simulink model "order_reduction_model"  (R2021a)
settings: Solver=FixedStepAuto  StartTime=0.0  StopTime=conf.cycle.stop  FixedStep=conf.time.step  RelTol=1e-3
InitFcn:
  | full_model_init;
  | load([pwd '\Data\pca_results.mat']);
values from neighbouring files (symbols this model uses):
  A = AB(1:10,:)    [order_reduction_script.m]
  B = AB(11:12,:)    [order_reduction_script.m]
  cellsP = conf.cells.p    [full_model_init.m]
  cellsS = conf.modules.x*conf.modules.y*conf.cells.s    [full_model_init.m]
  cellsTot = cellsS*cellsP    [full_model_init.m]
  elecC1 = C1_matrix*elecCellCap/cellCapGiant    [full_model_init.m]
  elecCellCap = 60    [full_model_init.m]
  elecInitSOC = (1 - variation)*socAve + 2*variation*socAve*rand(cellsS,cellsP)    [full_model_init.m]
  elecLoadDenomInds = 0    [full_model_init.m]
  elecLoadTerm12Inds = 0    [full_model_init.m]
  elecLoadTerm1Inds = 0    [full_model_init.m]
  elecLoadTerm2Inds = 0    [full_model_init.m]
  elecLoadTerm3Inds = 0    [full_model_init.m]
  elecOCV = Em_matrix    [full_model_init.m]
  elecR0 = R1_matrix*cellCapGiant/elecCellCap    [full_model_init.m]
  elecR1 = R2_matrix*cellCapGiant/elecCellCap    [full_model_init.m]
  elecSOCBreak = SOC_breakpoints    [full_model_init.m]
  elecTempBreak = Temp_breakpoints    [full_model_init.m]
  maxFlow = min([maxFlowX maxFlowY])    [full_model_init.m]
  mdotDistX = mdotDistX*flowMult    [full_model_init.m]
  mdotDistY = mdotDistY*flowMult    [full_model_init.m]
  tempAmb = conf.bound.amb    [full_model_init.m]    (also in order_reduction_script.m = data.tempAmb)
  tempTarget = 25    [full_model_init.m]
  thermCellVols = (thermHeatInds ~= 0)    [full_model_init.m]
  thermHeatCellToVol = 1/(conf.regions.l*conf.regions.w*conf.regions.t)    [full_model_init.m]
  thermTempInds = zeros(conf.regions.l*conf.regions.w*conf.regions.t,1,cellsS*cellsP)    [full_model_init.m]
  vehAf = 3.15    [full_model_init.m]
  vehCd = 0.28    [full_model_init.m]
  vehM = 2565    [full_model_init.m]
  vehPowerMult = modelEnergy/packEnergy    [full_model_init.m]
undefined symbols (not defined in the file or in its folder): conf, loadDenomInds, loadTerm12Inds, loadTerm1Inds, loadTerm2Inds, loadTerm3Inds, parallelCells, radAirVelBreakPoints, radCoolFlowBreakPoints, radNomFlowMatrix, refAirVelBreakPoints, refCoolFlowBreakPoints, refCoolInTempBreakPoints, refTempOutMatrix, seriesCells, thermDims
libraries: visionstatistics x1
settings Model: NumberOfSteps=100  Creator=sjtho  LastModifiedBy=sjtho
settings OptimizationCC: OptimizeBlockIOStorage=off  OptimizeDataStoreBuffers=off  BusAssignmentInplaceUpdate=off
settings DebuggingCC: UniqueDataStoreMsg=error  SFUnexpectedBacktrackingDiag=warning  SFNoUnconditionalDefaultTransitionDiag=warning
settings RTWCC: GenerateReport=on  BuildConfiguration=Debug  LaunchReport=on
settings CodeAppCC: ForceParamTrailComments=on  MATLABSourceComments=on  EnableCustomComments=on
settings GRTTargetCC: CombineSignalStateStructs=on  SupportVariableSizeSignals=on  MultiInstanceErrorCode=Warning

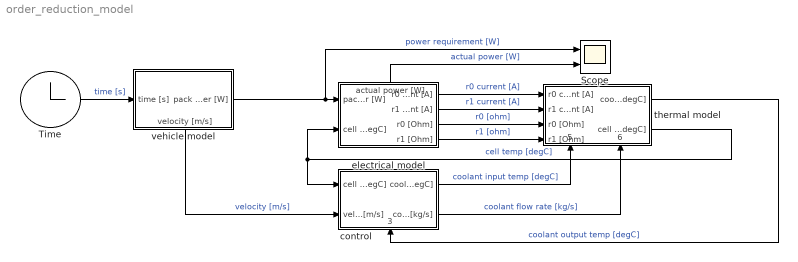
== system order_reduction_model ==
  Scope : Scope  NumInputPorts=2
  Time : Clock
  control : Subsystem
      settings: PortSchema="{\"entries\":[{\"content\":{\"sides\":[{\"content\":{\"connectorIds\":[\"In1\",\"In2\"]},\"type\":\"ConnectorPlacement.EquallySpacedRectSide\",\"uuid\":\"22f80eaa-bb46-4281-9ec1-3970c1bac2a3\"},{\"content\":{\"connectorIds\":[\"Out1\",\"Out2\"],\"side\":\"RIGHT\"},\"type\":\"ConnectorPlacement.EquallySpacedRectSide\",\"uuid\":\"e76f71c5-d41f-442d-b655-b3bc32395443\"},{\"content\":{\"connectorIds\":[],\"side\":\"TOP\"},\"type\":\"ConnectorPlacement.EquallySpacedRectSide\",\"uuid\":\"e3a9d903-5780-49ee-b4b3-f001d4a3722b\"},{\"content\":{\"connectorIds\":[\"In3\"],\"side\":\"BOTTOM\"},\"type\":\"ConnectorPlacement.EquallySpacedRectSide\",\"uuid\":\"8a36595f-00ae-4362-a59c-271e32328d9e\"}]},\"type\":\"ConnectorPlacement.EquallySpacedConnector\",\"uuid\":\"d37af0d9-ec54-4f0d-b375-47d72f1b804c\"}],\"packageUris\":[\"http://schema.mathworks.com/mf0/Connector/R2020b\"],\"version\":\"1.0\"}"
      mask Display: disp(['Control and ' newline 'Cooling'])
  electrical model : Subsystem
      settings: PortSchema="{\"entries\":[{\"content\":{\"sides\":[{\"content\":{\"connectorIds\":[\"In1\",\"In2\"]},\"type\":\"ConnectorPlacement.EquallySpacedRectSide\",\"uuid\":\"4f52e6ae-bc3b-4951-b08d-fa2762ef8feb\"},{\"content\":{\"connectorIds\":[\"Out1\",\"Out2\",\"Out3\",\"Out4\"],\"side\":\"RIGHT\"},\"type\":\"ConnectorPlacement.EquallySpacedRectSide\",\"uuid\":\"4046dfc3-1b24-4486-8fe3-cced4e699fd9\"},{\"content\":{\"connectorIds\":[\"Out5\"],\"side\":\"TOP\"},\"type\":\"ConnectorPlacement.EquallySpacedRectSide\",\"uuid\":\"da108a30-fb00-422c-8122-750755c2660a\"}]},\"type\":\"ConnectorPlacement.EquallySpacedConnector\",\"uuid\":\"4753e952-e769-49fa-907f-6d09e5e535ba\"}],\"packageUris\":[\"http://schema.mathworks.com/mf0/Connector/R2020b\"],\"version\":\"1.0\"}"
      mask Display: disp('Electrical Model')
  thermal model : Subsystem
      settings: PortSchema="{\"entries\":[{\"content\":{\"sides\":[{\"content\":{\"connectorIds\":[\"In1\",\"In2\",\"In3\",\"In4\"]},\"type\":\"ConnectorPlacement.EquallySpacedRectSide\",\"uuid\":\"85abd361-fdf9-4e50-9692-c6cfc682c3ac\"},{\"content\":{\"connectorIds\":[\"Out1\",\"Out2\"],\"side\":\"RIGHT\"},\"type\":\"ConnectorPlacement.EquallySpacedRectSide\",\"uuid\":\"50be5dc9-6285-4d3d-a0f1-610cf70c20d6\"},{\"content\":{\"connectorIds\":[],\"side\":\"TOP\"},\"type\":\"ConnectorPlacement.EquallySpacedRectSide\",\"uuid\":\"1bb98c42-8893-43bf-953b-d262aeaa61fe\"},{\"content\":{\"connectorIds\":[\"In5\",\"In6\"],\"side\":\"BOTTOM\"},\"type\":\"ConnectorPlacement.EquallySpacedRectSide\",\"uuid\":\"83d18484-4c30-41fd-9096-006931d5d21f\"}]},\"type\":\"ConnectorPlacement.EquallySpacedConnector\",\"uuid\":\"8afb65a4-2410-4c66-9cd3-3c36ab441c83\"}],\"packageUris\":[\"http://schema.mathworks.com/mf0/Connector/R2020b\"],\"version\":\"1.0\"}"
      mask Display: disp('Thermal Model')
  vehicle model : Subsystem
      settings: PortSchema="{\"entries\":[{\"content\":{\"sides\":[{\"content\":{\"connectorIds\":[\"In1\"]},\"type\":\"ConnectorPlacement.EquallySpacedRectSide\",\"uuid\":\"cf313784-55fc-4068-b83a-27fead484f77\"},{\"content\":{\"connectorIds\":[\"Out1\"],\"side\":\"RIGHT\"},\"type\":\"ConnectorPlacement.EquallySpacedRectSide\",\"uuid\":\"2b8b7e96-e7dc-4089-926d-80148fade29f\"},{\"content\":{\"connectorIds\":[],\"side\":\"TOP\"},\"type\":\"ConnectorPlacement.EquallySpacedRectSide\",\"uuid\":\"332287a3-327f-4bf8-9290-89809e483fea\"},{\"content\":{\"connectorIds\":[\"Out2\"],\"side\":\"BOTTOM\"},\"type\":\"ConnectorPlacement.EquallySpacedRectSide\",\"uuid\":\"f07f6670-fe7e-40c0-9cd8-41a00d5f5993\"}]},\"type\":\"ConnectorPlacement.EquallySpacedConnector\",\"uuid\":\"6bd39f86-8f76-4883-86c4-8a861857bd9f\"}],\"packageUris\":[\"http://schema.mathworks.com/mf0/Connector/R2020b\"],\"version\":\"1.0\"}"
      mask Display: disp('Vehicle Model')
  wires:
  Time/1 -> vehicle model/1(time [s])  "time [s]"
  vehicle model/1(pack power [W]) -> Scope/1, electrical model/1(pack power [W])  "power requirement [W]"
  control/1(coolant input temp [degC]) -> thermal model/5(coolant input temp [degC])  "coolant input temp [degC]"
  thermal model/1(coolant output temp [degC]) -> control/3(coolant output temp [degC])  "coolant output temp [degC]"
  electrical model/1(r0 current [A]) -> thermal model/1(r0 current [A])  "r0 current [A]"
  electrical model/2(r1 current [A]) -> thermal model/2(r1 current [A])  "r1 current [A]"
  electrical model/3(r0 [Ohm]) -> thermal model/3(r0 [Ohm])  "r0 [ohm]"
  electrical model/4(r1 [Ohm]) -> thermal model/4(r1 [Ohm])  "r1 [ohm]"
  thermal model/2(cell temp [degC]) -> electrical model/2(cell temp [degC]), control/1(cell temp [degC])  "cell temp [degC]"
  electrical model/5(actual power [W]) -> Scope/2  "actual power [W]"
  vehicle model/2(velocity [m/s]) -> control/2(velocity [m/s])  "velocity [m/s]"
  control/2(coolant flow rate [kg/s]) -> thermal model/6(coolant flow rate [kg/s])  "coolant flow rate [kg/s]"

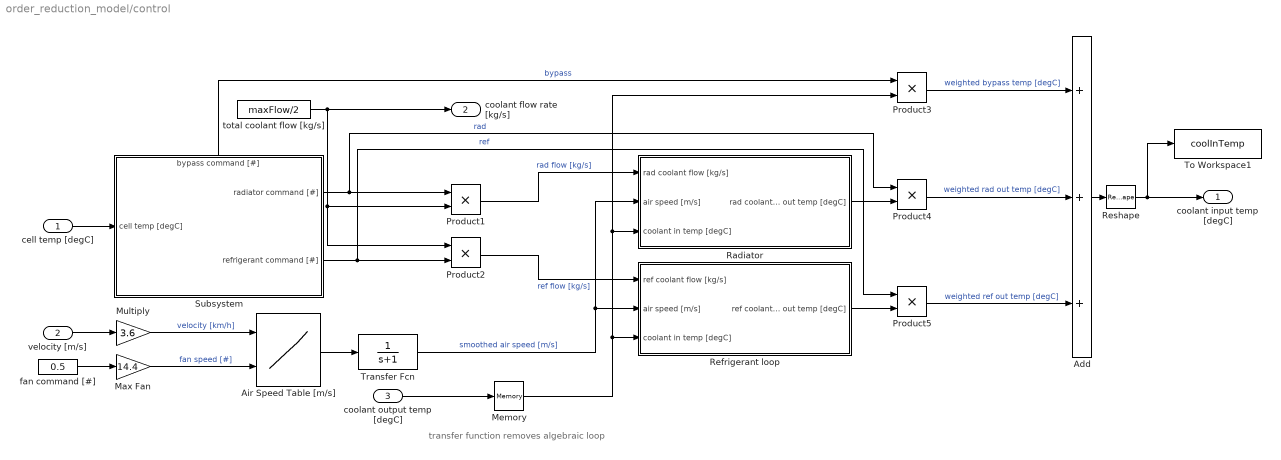
== system order_reduction_model/control ==
  note: transfer function removes algebraic loop
  cell temp [degC] : Inport
  velocity [m/s] : Inport  Port=2
  coolant output temp [degC] : Inport  Port=3
  Add : Sum  Inputs=+++
  Air Speed Table [m/s] : Lookup_n-D  BreakpointsForDimension1=[0 40 90 110 150 180 198]  BreakpointsForDimension2=[0 14.4]  IndexSearchMethod=Linear search  BeginIndexSearchUsingPreviousIndexResult=on  Table=[0 0.8 2.2 2.7 3.6 4.1 4.6; 1.5 2.3 3.2 3.5 4.3 4.8 5.1]'  InternalRulePriority=Speed  RndMeth=Simplest  InputSameDT=on
      settings: InputPortMap=u0,u1
  Max Fan : Gain  Gain=14.4
  Memory : Memory  InitialCondition=tempAmb + conf.bound.initBias
  Multiply : Gain  Gain=3.6
  Product{1..5} (5 alike) : Product
  Radiator : Subsystem
  Refrigerant loop : Subsystem
  Reshape : Reshape  OutputDimensionality=Customize  OutputDimensions=1
  Subsystem : Subsystem
      settings: PortSchema="{\"entries\":[{\"content\":{\"sides\":[{\"content\":{\"connectorIds\":[\"In1\"]},\"type\":\"ConnectorPlacement.EquallySpacedRectSide\",\"uuid\":\"39caf9d2-37e9-4ddb-8f89-28cdec2ac0f1\"},{\"content\":{\"connectorIds\":[\"Out1\",\"Out2\"],\"side\":\"RIGHT\"},\"type\":\"ConnectorPlacement.EquallySpacedRectSide\",\"uuid\":\"3cbc02da-b039-4e1d-b42e-efc08ec78021\"},{\"content\":{\"connectorIds\":[\"Out3\"],\"side\":\"TOP\"},\"type\":\"ConnectorPlacement.EquallySpacedRectSide\",\"uuid\":\"b4b3f97e-dd64-49e3-8c52-9947fb1a0732\"}]},\"type\":\"ConnectorPlacement.EquallySpacedConnector\",\"uuid\":\"4860c07b-2c7d-4cd4-976e-5c2ba4e5db64\"}],\"packageUris\":[\"http://schema.mathworks.com/mf0/Connector/R2020b\"],\"version\":\"1.0\"}"
  To Workspace1 : ToWorkspace  VariableName=coolInTemp  SaveFormat=Timeseries  SampleTime=conf.time.sample
  Transfer Fcn : TransferFcn  Denominator=[1 1]
  fan command [#] : Constant  Value=0.5
  total coolant flow [kg/s] : Constant  Value=maxFlow/2
  coolant input temp [degC] : Outport
  coolant flow rate [kg/s] : Outport  Port=2
  wires:
  Max Fan/1 -> Air Speed Table [m/s]/2  "fan speed [#]"
  velocity [m/s]/1 -> Multiply/1
  fan command [#]/1 -> Max Fan/1
  Multiply/1 -> Air Speed Table [m/s]/1  "velocity [km/h]"
  Air Speed Table [m/s]/1 -> Transfer Fcn/1
  cell temp [degC]/1 -> Subsystem/1(cell temp [degC])
  Subsystem/1(radiator command [#]) -> Product1/1, Product4/1  "rad"
  Subsystem/2(refrigerant command [#]) -> Product5/1, Product2/2  "ref"
  Product1/1 -> Radiator/1(rad coolant flow [kg/s])  "rad flow [kg/s]"
  Product2/1 -> Refrigerant loop/1(ref coolant flow [kg/s])  "ref flow [kg/s]"
  Transfer Fcn/1 -> Radiator/2(air speed [m/s]), Refrigerant loop/2(air speed [m/s])  "smoothed air speed [m/s]"
  coolant output temp [degC]/1 -> Memory/1
  Refrigerant loop/1(ref coolant out temp [degC]) -> Product5/2
  Radiator/1(rad coolant out temp [degC]) -> Product4/2
  Product4/1 -> Add/2  "weighted rad out temp [degC]"
  Product5/1 -> Add/3  "weighted ref out temp [degC]"
  Product3/1 -> Add/1  "weighted bypass temp [degC]"
  Subsystem/3(bypass command [#]) -> Product3/1  "bypass"
  total coolant flow [kg/s]/1 -> Product2/1, Product1/2, coolant flow rate [kg/s]/1
  Memory/1 -> Product3/2, Radiator/3(coolant in temp [degC]), Refrigerant loop/3(coolant in temp [degC])
  Add/1 -> Reshape/1
  Reshape/1 -> To Workspace1/1, coolant input temp [degC]/1

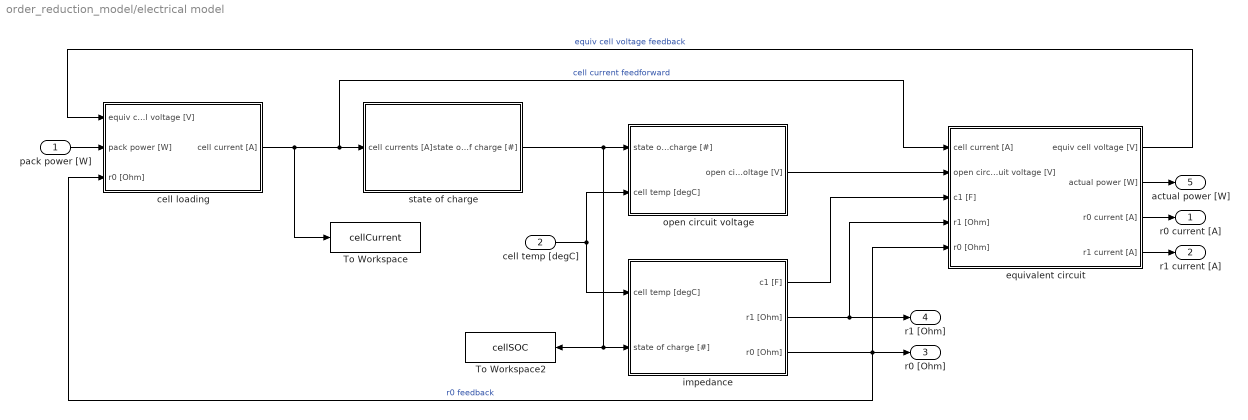
== system order_reduction_model/electrical model ==
  pack power [W] : Inport
  cell temp [degC] : Inport  Port=2
  To Workspace : ToWorkspace  VariableName=cellCurrent  SaveFormat=Timeseries  SampleTime=conf.time.sample
  To Workspace2 : ToWorkspace  VariableName=cellSOC  SaveFormat=Timeseries  SampleTime=conf.time.sample
  cell loading : Subsystem
  equivalent circuit : Subsystem
  impedance : Subsystem
  open circuit voltage : Subsystem
  state of charge : Subsystem
  r0 current [A] : Outport
  r1 current [A] : Outport  Port=2
  r0 [Ohm] : Outport  Port=3
  r1 [Ohm] : Outport  Port=4
  actual power [W] : Outport  Port=5
  wires:
  cell loading/1(cell current [A]) -> To Workspace/1, state of charge/1(cell currents [A]), equivalent circuit/1(cell current [A])  "cell current feedforward"
  cell temp [degC]/1 -> open circuit voltage/2(cell temp [degC]), impedance/1(cell temp [degC])
  state of charge/1(state of charge [#]) -> open circuit voltage/1(state of charge [#]), To Workspace2/1, impedance/2(state of charge [#])
  open circuit voltage/1(open circuit voltage [V]) -> equivalent circuit/2(open circuit voltage [V])
  equivalent circuit/2(actual power [W]) -> actual power [W]/1
  equivalent circuit/3(r0 current [A]) -> r0 current [A]/1
  equivalent circuit/4(r1 current [A]) -> r1 current [A]/1
  equivalent circuit/1(equiv cell voltage [V]) -> cell loading/1(equiv cell voltage [V])  "equiv cell voltage feedback"
  pack power [W]/1 -> cell loading/2(pack power [W])
  impedance/1(c1 [F]) -> equivalent circuit/3(c1 [F])
  impedance/2(r1 [Ohm]) -> r1 [Ohm]/1, equivalent circuit/4(r1 [Ohm])
  impedance/3(r0 [Ohm]) -> r0 [Ohm]/1, cell loading/3(r0 [Ohm]), equivalent circuit/5(r0 [Ohm])  "r0 feedback"

== system order_reduction_model/thermal model ==
  r0 current [A] : Inport
  r1 current [A] : Inport  Port=2
  r0 [Ohm] : Inport  Port=3
  r1 [Ohm] : Inport  Port=4
  coolant input temp [degC] : Inport  Port=5
  coolant flow rate [kg/s] : Inport  Port=6
  Subsystem : Subsystem
      mask Display: disp('Coolant Output Temp');
  cell temp : Subsystem
      mask Display: disp('Cell Temp')
  heat generation : Subsystem
      mask Display: disp('Heat Generation')
  coolant output temp [degC] : Outport
  cell temp [degC] : Outport  Port=2
  wires:
  coolant input temp [degC]/1 -> cell temp/2(coolant input temp [degC])
  r0 current [A]/1 -> heat generation/1(r0 current [A])
  r1 current [A]/1 -> heat generation/2(r1 current [A])
  r0 [Ohm]/1 -> heat generation/3(r0 [Ohm])
  r1 [Ohm]/1 -> heat generation/4(r1 [Ohm])
  heat generation/1(total heat generation [W]) -> cell temp/1(net heat gain [W])  "total heat generation [W]"
  cell temp/1(cell temp [degC]) -> cell temp [degC]/1
  Subsystem/1(coolant output temp [degC]) -> coolant output temp [degC]/1
  cell temp/2(vol temp [degC]) -> Subsystem/2(volume temp [degC])  "volume temp [degC]"
  coolant flow rate [kg/s]/1 -> Subsystem/1(coolant flow rate [kg/s])

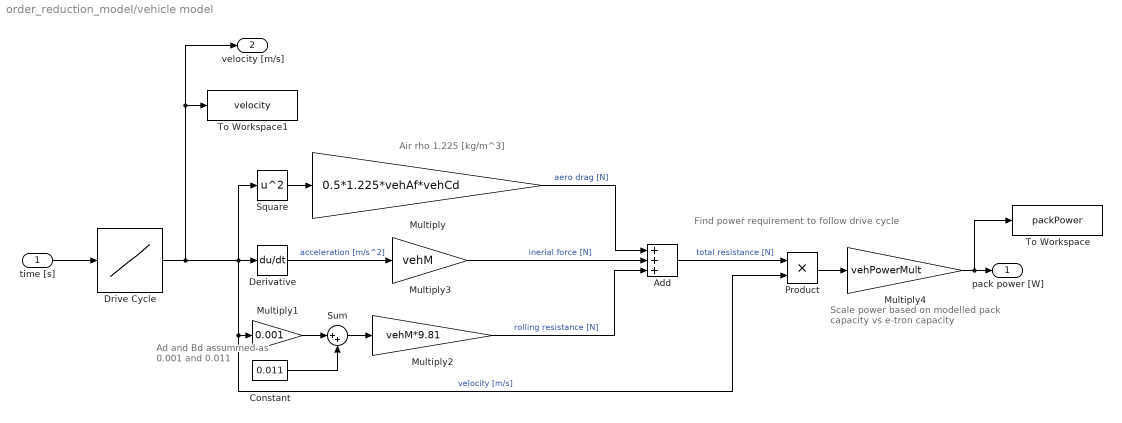
== system order_reduction_model/vehicle model ==
  note: Scale power based on modelled pack capacity vs e-tron capacity
  note: Ad and Bd assummed as 0.001 and 0.011
  note: Air rho 1.225 [kg/m^3]
  note: Find power requirement to follow drive cycle
  time [s] : Inport
  Add : Sum  Inputs=+++
  Constant : Constant  Value=0.011
  Derivative : Derivative
  Drive Cycle : Lookup_n-D  NumberOfTableDimensions=1  BreakpointsForDimension1=conf.cycle.time  Table=conf.cycle.vel  InterpMethod=Cubic spline  InternalRulePriority=Speed  RndMeth=Simplest  InputSameDT=on
  Multiply : Gain  Gain=0.5*1.225*vehAf*vehCd
  Multiply1 : Gain  Gain=0.001
  Multiply2 : Gain  Gain=vehM*9.81
  Multiply3 : Gain  Gain=vehM
  Multiply4 : Gain  Gain=vehPowerMult
  Product : Product
  Square : Math  Operator=square  SaturateOnIntegerOverflow=on
  Sum : Sum  Inputs=|++
  To Workspace : ToWorkspace  VariableName=packPower  SaveFormat=Timeseries  SampleTime=conf.time.sample
  To Workspace1 : ToWorkspace  VariableName=velocity  SaveFormat=Timeseries  SampleTime=conf.time.sample
  pack power [W] : Outport
  velocity [m/s] : Outport  Port=2
  wires:
  time [s]/1 -> Drive Cycle/1
  Multiply/1 -> Add/1  "aero drag [N]"
  Drive Cycle/1 -> velocity [m/s]/1, To Workspace1/1, Derivative/1, Multiply1/1, Product/2, Square/1  "velocity [m/s]"
  Add/1 -> Product/1  "total resistance [N]"
  Multiply3/1 -> Add/2  "inerial force [N]"
  Square/1 -> Multiply/1
  Multiply1/1 -> Sum/1
  Derivative/1 -> Multiply3/1  "acceleration [m/s^2]"
  Sum/1 -> Multiply2/1
  Constant/1 -> Sum/2
  Multiply2/1 -> Add/3  "rolling resistance [N]"
  Product/1 -> Multiply4/1
  Multiply4/1 -> To Workspace/1, pack power [W]/1

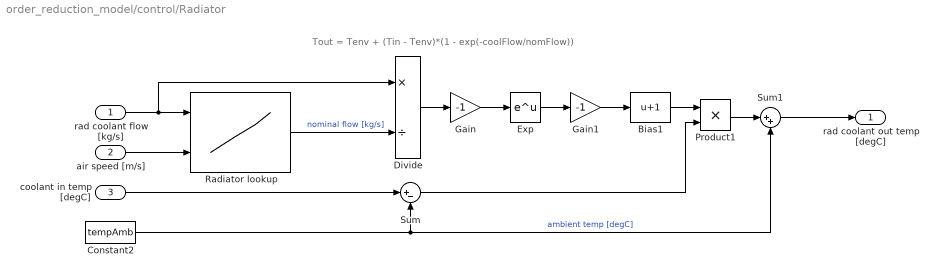
== system order_reduction_model/control/Radiator ==
  note: Tout = Tenv + (Tin - Tenv)*(1 - exp(-coolFlow/nomFlow))
  rad coolant flow [kg/s] : Inport
  air speed [m/s] : Inport  Port=2
  coolant in temp [degC] : Inport  Port=3
  Bias1 : Bias  Bias=1
  Constant2 : Constant  Value=tempAmb
  Divide : Product  Inputs=*/
  Exp : Math  SaturateOnIntegerOverflow=on
  Gain : Gain  Gain=-1
  Gain1 : Gain  Gain=-1
  Product1 : Product
  Radiator lookup : Lookup_n-D  BreakpointsForDimension1=radCoolFlowBreakPoints  BreakpointsForDimension2=radAirVelBreakPoints  BreakpointsForDimension3=refCoolInTempBreakPoints  Table=radNomFlowMatrix  InternalRulePriority=Speed  RndMeth=Simplest  InputSameDT=on
      settings: InputPortMap=u0,u1
  Sum : Sum  Inputs=|+-
  Sum1 : Sum  Inputs=|++
  rad coolant out temp [degC] : Outport
  wires:
  Radiator lookup/1 -> Divide/2  "nominal flow [kg/s]"
  Product1/1 -> Sum1/1
  rad coolant flow [kg/s]/1 -> Divide/1, Radiator lookup/1
  air speed [m/s]/1 -> Radiator lookup/2
  Divide/1 -> Gain/1
  Gain/1 -> Exp/1
  Exp/1 -> Gain1/1
  Gain1/1 -> Bias1/1
  Bias1/1 -> Product1/1
  coolant in temp [degC]/1 -> Sum/1
  Constant2/1 -> Sum1/2, Sum/2  "ambient temp [degC]"
  Sum/1 -> Product1/2
  Sum1/1 -> rad coolant out temp [degC]/1

== system order_reduction_model/control/Refrigerant loop ==
  ref coolant flow [kg/s] : Inport
  air speed [m/s] : Inport  Port=2
  coolant in temp [degC] : Inport  Port=3
  Refrigerant Loop : Lookup_n-D  NumberOfTableDimensions=3  BreakpointsForDimension1=refCoolFlowBreakPoints  BreakpointsForDimension2=refAirVelBreakPoints  BreakpointsForDimension3=refCoolInTempBreakPoints  Table=refTempOutMatrix  InternalRulePriority=Speed  RndMeth=Simplest  InputSameDT=on
      settings: InputPortMap=u0,u1,u2
  ref coolant out temp [degC] : Outport
  wires:
  air speed [m/s]/1 -> Refrigerant Loop/2
  coolant in temp [degC]/1 -> Refrigerant Loop/3
  Refrigerant Loop/1 -> ref coolant out temp [degC]/1
  ref coolant flow [kg/s]/1 -> Refrigerant Loop/1

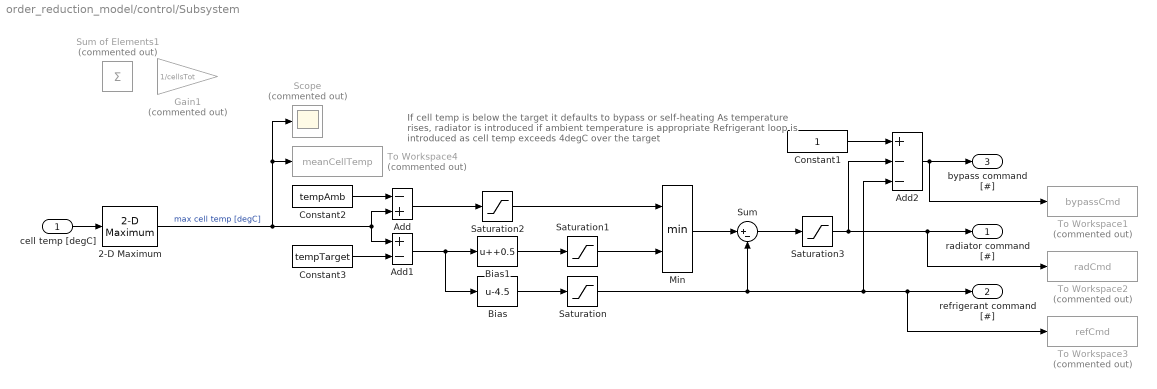
== system order_reduction_model/control/Subsystem ==
  note: If cell temp is below the target it defaults to bypass or self-heating
      | As temperature rises, radiator is introduced if ambient temperature is appropriate
      | Refrigerant loop is introduced as cell temp exceeds 4degC over the target
  cell temp [degC] : Inport
  2-D Maximum : visionstatistics/2-D Maximum  fcn=Value  reset=None  indexBase=One  operateOver=Entire input  Dimension=1  colComp=on  operation=maximum  accumLastDataTypeStr=Inherit: Same as product output  roiEnable=off  roiType=Rectangles  roiPortion=Entire ROI  roiOutput=Individual statistics for each ROI  roiFlag=off  roundingMode=Floor  overflowMode=off  accumDataTypeStr=Inherit: Same as product output
      settings: SourceProductBaseCode=VP
  Add : Sum  Inputs=-+
  Add1 : Sum  Inputs=+-
  Add2 : Sum  Inputs=+--
  Bias : Bias  Bias=-4.5
  Bias1 : Bias  Bias=+0.5
  Constant1 : Constant
  Constant2 : Constant  Value=tempAmb
  Constant3 : Constant  Value=tempTarget
  Gain1 : Gain  Commented=on  Gain=1/cellsTot
  Min : MinMax  Inputs=2
  Saturation{,1..3} (4 alike) : Saturate  UpperLimit=1  LowerLimit=0
  Scope : Scope  Commented=on
  Sum : Sum  Inputs=|+-
  Sum of Elements1 : Sum  Commented=on  Inputs=+
  To Workspace1 : ToWorkspace  Commented=on  VariableName=bypassCmd  SaveFormat=Timeseries  SampleTime=conf.time.sample
  To Workspace2 : ToWorkspace  Commented=on  VariableName=radCmd  SaveFormat=Timeseries  SampleTime=conf.time.sample
  To Workspace3 : ToWorkspace  Commented=on  VariableName=refCmd  SaveFormat=Timeseries  SampleTime=conf.time.sample
  To Workspace4 : ToWorkspace  Commented=on  VariableName=meanCellTemp  SaveFormat=Timeseries  SampleTime=conf.time.sample
  radiator command [#] : Outport
  refrigerant command [#] : Outport  Port=2
  bypass command [#] : Outport  Port=3
  wires:
  cell temp [degC]/1 -> 2-D Maximum/1
  2-D Maximum/1 -> Scope/1, To Workspace4/1, Add1/1, Add/2  "max cell temp [degC]"
  Constant3/1 -> Add1/2
  Constant2/1 -> Add/1
  Add1/1 -> Bias1/1, Bias/1
  Bias/1 -> Saturation/1
  Saturation/1 -> Add2/3, To Workspace3/1, refrigerant command [#]/1, Sum/2
  Add/1 -> Saturation2/1
  Bias1/1 -> Saturation1/1
  Saturation2/1 -> Min/1
  Saturation1/1 -> Min/2
  Min/1 -> Sum/1
  Sum/1 -> Saturation3/1
  Saturation3/1 -> To Workspace2/1, radiator command [#]/1, Add2/2
  Constant1/1 -> Add2/1
  Add2/1 -> To Workspace1/1, bypass command [#]/1

== system order_reduction_model/electrical model/cell loading ==
  note: Using if statement to calculate cell current in the correct way. This varies based on the number of parallel cells
  note: Old function using matlab block, replace this with simulink only for speed
  note: Solving quadratic equation for cell current using the smaller solution
      | and then splitting this value between all the cells
  equiv cell voltage [V] : Inport
  pack power [W] : Inport  Port=2
  r0 [Ohm] : Inport  Port=3
  Cell Loading Function : MATLAB Function  TreatAsAtomicUnit=on
  Cell Loading Function2 : MATLAB Function  Commented=on  TreatAsAtomicUnit=on
  Pack current : Subsystem
  Pack voltage and resistance : Subsystem
  Reshape : Reshape  OutputDimensionality=Customize  OutputDimensions=1
  cell current [A] : Outport
  wires:
  r0 [Ohm]/1 -> Cell Loading Function/3(r0Mat), Pack voltage and resistance/2(r0 [Ohm])
  Pack voltage and resistance/1(pack thevenin voltage [V]) -> Pack current/1(pack thevenin voltage [V])
  Pack voltage and resistance/2(pack thevenin resistance [Ohm]) -> Pack current/2(pack thevenin resistance [Ohm])
  pack power [W]/1 -> Pack current/3(pack power [W])
  equiv cell voltage [V]/1 -> Cell Loading Function/1(veqMat), Pack voltage and resistance/1(equiv cell voltage [V])
  Cell Loading Function/1(cellCurrent) -> cell current [A]/1
  Reshape/1 -> Cell Loading Function/2(ibat)
  Pack current/1(pack current [A]) -> Reshape/1

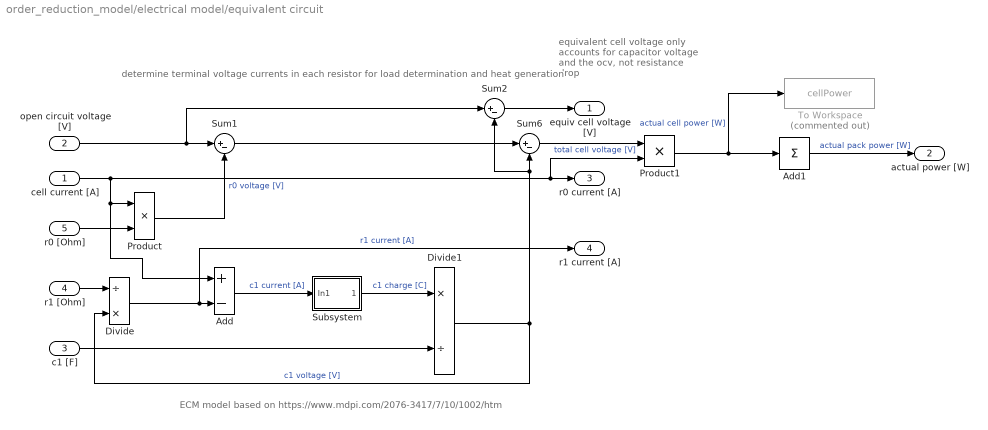
== system order_reduction_model/electrical model/equivalent circuit ==
  note: equivalent cell voltage only accounts for capacitor voltage and the ocv, not resistance drop
  note: determine terminal voltage currents in each resistor for load determination and heat generation
  note: ECM model based on https://www.mdpi.com/2076-3417/7/10/1002/htm
  cell current [A] : Inport
  open circuit voltage [V] : Inport  Port=2
  c1 [F] : Inport  Port=3
  r1 [Ohm] : Inport  Port=4
  r0 [Ohm] : Inport  Port=5
  Add : Sum  Inputs=+-
  Add1 : Sum  Inputs=+
  Divide : Product  Inputs=/*
  Divide1 : Product  Inputs=*/
  Product : Product
  Product1 : Product
  Subsystem : Subsystem
      mask Display: disp('DT Int');
  Sum1 : Sum  Inputs=|+-
  Sum2 : Sum  Inputs=|+-
  Sum6 : Sum  Inputs=|+-
  To Workspace : ToWorkspace  Commented=on  VariableName=cellPower  SaveFormat=Timeseries  SampleTime=conf.time.sample
  equiv cell voltage [V] : Outport
  actual power [W] : Outport  Port=2
  r0 current [A] : Outport  Port=3
  r1 current [A] : Outport  Port=4
  wires:
  Add/1 -> Subsystem/1(In1)  "c1 current [A]"
  Subsystem/1(Out1) -> Divide1/1  "c1 charge [C]"
  Divide/1 -> r1 current [A]/1, Add/2  "r1 current [A]"
  Sum1/1 -> Sum6/1
  Product/1 -> Sum1/2  "r0 voltage [V]"
  c1 [F]/1 -> Divide1/2
  Divide1/1 -> Divide/2, Sum2/2, Sum6/2  "c1 voltage [V]"
  open circuit voltage [V]/1 -> Sum2/1, Sum1/1
  cell current [A]/1 -> Product1/2, r0 current [A]/1, Product/1, Add/1
  r0 [Ohm]/1 -> Product/2
  r1 [Ohm]/1 -> Divide/1
  Sum2/1 -> equiv cell voltage [V]/1
  Sum6/1 -> Product1/1  "total cell voltage [V]"
  Product1/1 -> To Workspace/1, Add1/1  "actual cell power [W]"
  Add1/1 -> actual power [W]/1  "actual pack power [W]"

== system order_reduction_model/electrical model/impedance ==
  note: Impedence determination using 2D look-up table with state of charge and temperature
  cell temp [degC] : Inport
  state of charge [#] : Inport  Port=2
  Capacitance 1 : Lookup_n-D  BreakpointsForDimension1=elecTempBreak  BreakpointsForDimension2=elecSOCBreak  Table=elecC1  InternalRulePriority=Speed  RndMeth=Simplest  InputSameDT=on
      settings: InputPortMap=u0,u1
  Resistance 0 : Lookup_n-D  BreakpointsForDimension1=elecTempBreak  BreakpointsForDimension2=elecSOCBreak  Table=elecR0  InternalRulePriority=Speed  RndMeth=Simplest  InputSameDT=on
      settings: InputPortMap=u0,u1
  Resistance 1 : Lookup_n-D  BreakpointsForDimension1=elecTempBreak  BreakpointsForDimension2=elecSOCBreak  Table=elecR1  InternalRulePriority=Speed  RndMeth=Simplest  InputSameDT=on
      settings: InputPortMap=u0,u1
  c1 [F] : Outport
  r1 [Ohm] : Outport  Port=2
  r0 [Ohm] : Outport  Port=3
  wires:
  state of charge [#]/1 -> Resistance 0/2, Resistance 1/2, Capacitance 1/2  "SOC [#]"
  Resistance 0/1 -> r0 [Ohm]/1
  Resistance 1/1 -> r1 [Ohm]/1
  Capacitance 1/1 -> c1 [F]/1
  cell temp [degC]/1 -> Capacitance 1/1, Resistance 1/1, Resistance 0/1  "cell temp [degC]"

== system order_reduction_model/electrical model/open circuit voltage ==
  note: Open circuit voltage determination using 2D look-up table with state of charge and temperature
  state of charge [#] : Inport
  cell temp [degC] : Inport  Port=2
  Open Circuit Voltage : Lookup_n-D  BreakpointsForDimension1=elecTempBreak  BreakpointsForDimension2=elecSOCBreak  Table=elecOCV  InternalRulePriority=Speed  RndMeth=Simplest  InputSameDT=on
      settings: InputPortMap=u0,u1
  open circuit voltage [V] : Outport
  wires:
  state of charge [#]/1 -> Open Circuit Voltage/2
  Open Circuit Voltage/1 -> open circuit voltage [V]/1
  cell temp [degC]/1 -> Open Circuit Voltage/1

== system order_reduction_model/electrical model/state of charge ==
  note: -1 as positive current in the model is discharge
  cell currents [A] : Inport
  Multiply : Gain  Gain=1/3600
  Multiply1 : Gain  Gain=-1/elecCellCap
  Subsystem : Subsystem
      mask Display: disp('DT Int');
  state of charge [#] : Outport
  wires:
  cell currents [A]/1 -> Multiply/1  "current [A]"
  Multiply1/1 -> Subsystem/1(In1)  "discharge normalised [#]"
  Multiply/1 -> Multiply1/1  "current [Hourly]"
  Subsystem/1(Out1) -> state of charge [#]/1  "soc [#]"

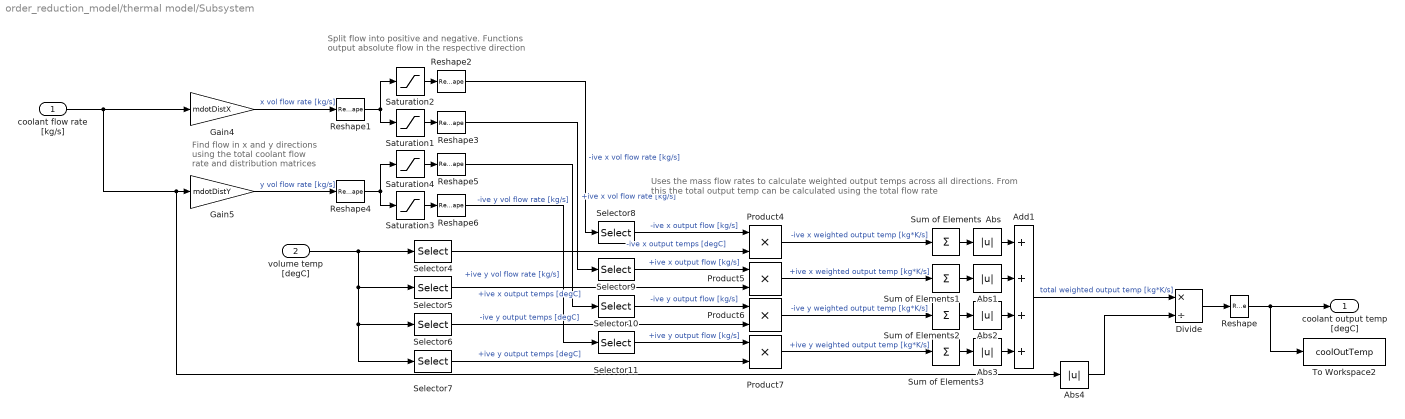
== system order_reduction_model/thermal model/Subsystem ==
  note: Find flow in x and y directions using the total coolant flow rate and distribution matrices
  note: Uses the mass flow rates to calculate weighted output temps across all directions. From this the total output temp can be calculated using the total flow rate
  note: Split flow into positive and negative. Functions output absolute flow in the respective direction
  coolant flow rate [kg/s] : Inport
  volume temp [degC] : Inport  Port=2
  Abs{,1..4} (5 alike) : Abs
  Add1 : Sum  Inputs=++++
  Divide : Product  Inputs=*/
  Gain4 : Gain  Gain=mdotDistX
  Gain5 : Gain  Gain=mdotDistY
  Product{4..7} (4 alike) : Product
  Reshape : Reshape  OutputDimensionality=Customize  OutputDimensions=1
  Reshape1 : Reshape  OutputDimensionality=Customize  OutputDimensions=thermDims(1)*thermDims(2)*thermDims(3)
  Reshape{2..3,5..6} (4 alike) : Reshape  OutputDimensionality=Customize  OutputDimensions=thermDims
  Reshape4 : Reshape  OutputDimensionality=Customize  OutputDimensions=thermDims(1)*thermDims(2)*thermDims(3)
  Saturation1 : Saturate  UpperLimit=inf  LowerLimit=0
  Saturation2 : Saturate  UpperLimit=0  LowerLimit=-inf
  Saturation3 : Saturate  UpperLimit=inf  LowerLimit=0
  Saturation4 : Saturate  UpperLimit=0  LowerLimit=-inf
  Selector10 : Selector  NumberOfDimensions=3  InputPortWidth=3  IndexOptions=Select all,Index vector (dialog),Select all  Indices=1,1,1:thermDims(3)  OutputSizes=1,1,1
  Selector11 : Selector  NumberOfDimensions=3  InputPortWidth=3  IndexOptions=Select all,Index vector (dialog),Select all  Indices=thermDims(1) + 1,thermDims(2),1:thermDims(3)  OutputSizes=1,1,1
  Selector4 : Selector  NumberOfDimensions=3  InputPortWidth=3  IndexOptions=Index vector (dialog),Select all,Select all  Indices=1,1:thermDims(2),1:thermDims(3)  OutputSizes=1,1,1
  Selector5 : Selector  NumberOfDimensions=3  InputPortWidth=3  IndexOptions=Index vector (dialog),Select all,Select all  Indices=thermDims(1),1:thermDims(2),1:thermDims(3)  OutputSizes=1,1,1
  Selector6 : Selector  NumberOfDimensions=3  InputPortWidth=3  IndexOptions=Select all,Index vector (dialog),Select all  Indices=1,1,1:thermDims(3)  OutputSizes=1,1,1
  Selector7 : Selector  NumberOfDimensions=3  InputPortWidth=3  IndexOptions=Select all,Index vector (dialog),Select all  Indices=thermDims(1) + 1,thermDims(2),1:thermDims(3)  OutputSizes=1,1,1
  Selector8 : Selector  NumberOfDimensions=3  InputPortWidth=3  IndexOptions=Index vector (dialog),Select all,Select all  Indices=1,1:thermDims(2),1:thermDims(3)  OutputSizes=1,1,1
  Selector9 : Selector  NumberOfDimensions=3  InputPortWidth=3  IndexOptions=Index vector (dialog),Select all,Select all  Indices=thermDims(1),1:thermDims(2),1:thermDims(3)  OutputSizes=1,1,1
  Sum of Elements{,1..3} (4 alike) : Sum  Inputs=+
  To Workspace2 : ToWorkspace  VariableName=coolOutTemp  SaveFormat=Timeseries  SampleTime=conf.time.sample
  coolant output temp [degC] : Outport
  wires:
  Saturation2/1 -> Reshape2/1
  volume temp [degC]/1 -> Selector6/1, Selector7/1, Selector5/1, Selector4/1
  Gain4/1 -> Reshape1/1  "x vol flow rate [kg/s]"
  Reshape3/1 -> Selector9/1  "+ive x vol flow rate [kg/s]"
  Selector7/1 -> Product7/2  "+ive y output temps [degC]"
  Saturation1/1 -> Reshape3/1
  Reshape1/1 -> Saturation1/1, Saturation2/1
  Reshape5/1 -> Selector10/1  "-ive y vol flow rate [kg/s]"
  Abs2/1 -> Add1/3
  Sum of Elements/1 -> Abs/1
  coolant flow rate [kg/s]/1 -> Abs4/1, Gain5/1, Gain4/1
  Product4/1 -> Sum of Elements/1  "-ive x weighted output temp [kg*K/s]"
  Abs3/1 -> Add1/4
  Reshape6/1 -> Selector11/1  "+ive y vol flow rate [kg/s]"
  Reshape2/1 -> Selector8/1  "-ive x vol flow rate [kg/s]"
  Product5/1 -> Sum of Elements1/1  "+ive x weighted output temp [kg*K/s]"
  Saturation3/1 -> Reshape6/1
  Selector9/1 -> Product5/1  "+ive x output flow [kg/s]"
  Selector5/1 -> Product5/2  "+ive x output temps [degC]"
  Selector10/1 -> Product6/1  "-ive y output flow [kg/s]"
  Product7/1 -> Sum of Elements3/1  "+ive y weighted output temp [kg*K/s]"
  Add1/1 -> Divide/1  "total weighted output temp [kg*K/s]"
  Saturation4/1 -> Reshape5/1
  Abs4/1 -> Divide/2
  Reshape4/1 -> Saturation4/1, Saturation3/1
  Gain5/1 -> Reshape4/1  "y vol flow rate [kg/s]"
  Selector4/1 -> Product4/2  "-ive x output temps [degC]"
  Sum of Elements3/1 -> Abs3/1
  Selector6/1 -> Product6/2  "-ive y output temps [degC]"
  Product6/1 -> Sum of Elements2/1  "-ive y weighted output temp [kg*K/s]"
  Selector11/1 -> Product7/1  "+ive y output flow [kg/s]"
  Divide/1 -> Reshape/1
  Abs1/1 -> Add1/2
  Selector8/1 -> Product4/1  "-ive x output flow [kg/s]"
  Sum of Elements1/1 -> Abs1/1
  Abs/1 -> Add1/1
  Sum of Elements2/1 -> Abs2/1
  Reshape/1 -> coolant output temp [degC]/1, To Workspace2/1

== system order_reduction_model/thermal model/cell temp ==
  note: Finite volume model swapped for state space model
  net heat gain [W] : Inport
  coolant input temp [degC] : Inport  Port=2
  State Space Model : Subsystem
  To Workspace : ToWorkspace  VariableName=volTemp  SaveFormat=Timeseries  SampleTime=conf.time.sample
  To Workspace1 : ToWorkspace  VariableName=cellTemp  SaveFormat=Timeseries  SampleTime=conf.time.sample
  map volume temp to cells : MATLAB Function  TreatAsAtomicUnit=on
  cell temp [degC] : Outport
  vol temp [degC] : Outport  Port=2
  wires:
  State Space Model/1(volume temp [degC]) -> To Workspace/1, vol temp [degC]/1, map volume temp to cells/1(volTemp)
  map volume temp to cells/1(cellTemp) -> To Workspace1/1, cell temp [degC]/1
  net heat gain [W]/1 -> State Space Model/1(heat generation [W])
  coolant input temp [degC]/1 -> State Space Model/2(coolant input temp [degC])

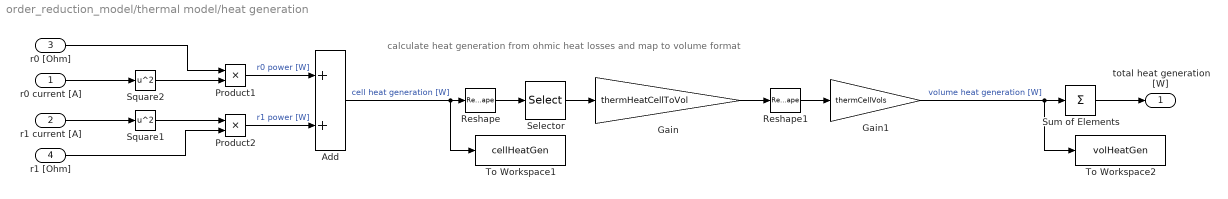
== system order_reduction_model/thermal model/heat generation ==
  note: calculate heat generation from ohmic heat losses and map to volume format
  r0 current [A] : Inport
  r1 current [A] : Inport  Port=2
  r0 [Ohm] : Inport  Port=3
  r1 [Ohm] : Inport  Port=4
  Add : Sum
  Gain : Gain  Gain=thermHeatCellToVol
  Gain1 : Gain  Gain=thermCellVols
  Product1 : Product
  Product2 : Product
  Reshape : Reshape
  Reshape1 : Reshape  OutputDimensionality=Customize  OutputDimensions=thermDims
  Selector : Selector  InputPortWidth=cellsS*cellsP  IndexOptions=Index vector (dialog)  Indices=thermHeatIndsNo0  OutputSizes=1
  Square1 : Math  Operator=square  SaturateOnIntegerOverflow=on
  Square2 : Math  Operator=square  SaturateOnIntegerOverflow=on
  Sum of Elements : Sum  Inputs=+
  To Workspace1 : ToWorkspace  VariableName=cellHeatGen  SaveFormat=Timeseries  SampleTime=conf.time.sample
  To Workspace2 : ToWorkspace  VariableName=volHeatGen  SaveFormat=Timeseries  SampleTime=conf.time.sample
  total heat generation [W] : Outport
  wires:
  Square1/1 -> Product2/1
  Product2/1 -> Add/2  "r1 power [W]"
  Square2/1 -> Product1/2
  r0 current [A]/1 -> Square2/1
  r1 current [A]/1 -> Square1/1
  r0 [Ohm]/1 -> Product1/1
  r1 [Ohm]/1 -> Product2/2
  Add/1 -> To Workspace1/1, Reshape/1  "cell heat generation [W]"
  Product1/1 -> Add/1  "r0 power [W]"
  Sum of Elements/1 -> total heat generation [W]/1
  Reshape/1 -> Selector/1
  Selector/1 -> Gain/1
  Gain/1 -> Reshape1/1
  Reshape1/1 -> Gain1/1
  Gain1/1 -> Sum of Elements/1, To Workspace2/1  "volume heat generation [W]"

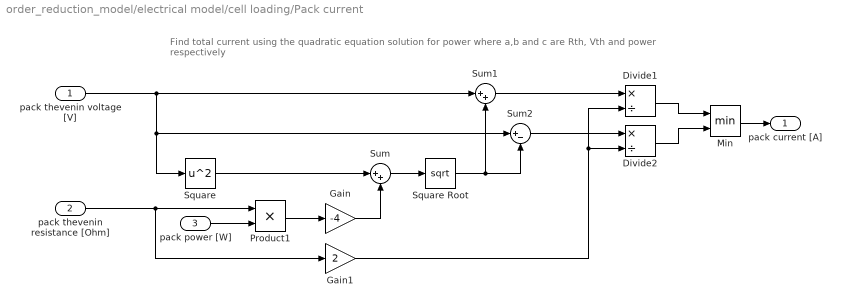
== system order_reduction_model/electrical model/cell loading/Pack current ==
  note: Find total current using the quadratic equation solution for power where a,b and c are Rth, Vth and power respectively
  pack thevenin voltage [V] : Inport
  pack thevenin resistance [Ohm] : Inport  Port=2
  pack power [W] : Inport  Port=3
  Divide1 : Product  Inputs=*/
  Divide2 : Product  Inputs=*/
  Gain : Gain  Gain=-4
  Gain1 : Gain  Gain=2
  Min : MinMax  Inputs=2
  Product1 : Product
  Square : Math  Operator=square  SaturateOnIntegerOverflow=on
  Square Root : Sqrt  SaturateOnIntegerOverflow=on
  Sum : Sum  Inputs=|++
  Sum1 : Sum  Inputs=|++
  Sum2 : Sum  Inputs=|+-
  pack current [A] : Outport
  wires:
  pack thevenin voltage [V]/1 -> Square/1, Sum2/1, Sum1/1
  Square/1 -> Sum/1
  Sum/1 -> Square Root/1
  pack thevenin resistance [Ohm]/1 -> Gain1/1, Product1/1
  Gain1/1 -> Divide2/2, Divide1/2
  Divide2/1 -> Min/2
  Square Root/1 -> Sum1/2, Sum2/2
  Sum2/1 -> Divide2/1
  Sum1/1 -> Divide1/1
  Divide1/1 -> Min/1
  Gain/1 -> Sum/2
  Product1/1 -> Gain/1
  pack power [W]/1 -> Product1/2
  Min/1 -> pack current [A]/1

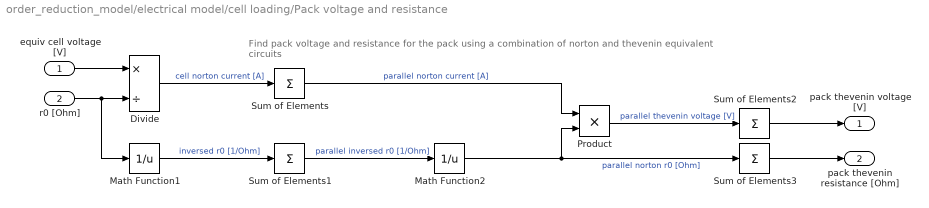
== system order_reduction_model/electrical model/cell loading/Pack voltage and resistance ==
  note: Find pack voltage and resistance for the pack using a combination of norton and thevenin equivalent circuits
  equiv cell voltage [V] : Inport
  r0 [Ohm] : Inport  Port=2
  Divide : Product  Inputs=*/
  Math Function1 : Math  Operator=reciprocal  SaturateOnIntegerOverflow=on
  Math Function2 : Math  Operator=reciprocal  SaturateOnIntegerOverflow=on
  Product : Product
  Sum of Elements : Sum  Inputs=+  CollapseMode=Specified dimension  CollapseDim=2
  Sum of Elements1 : Sum  Inputs=+  CollapseMode=Specified dimension  CollapseDim=2
  Sum of Elements2 : Sum  Inputs=+  CollapseMode=Specified dimension
  Sum of Elements3 : Sum  Inputs=+  CollapseMode=Specified dimension
  pack thevenin voltage [V] : Outport
  pack thevenin resistance [Ohm] : Outport  Port=2
  wires:
  Sum of Elements1/1 -> Math Function2/1  "parallel inversed r0 [1/Ohm]"
  r0 [Ohm]/1 -> Divide/2, Math Function1/1
  Divide/1 -> Sum of Elements/1  "cell norton current [A]"
  Sum of Elements/1 -> Product/1  "parallel norton current [A]"
  Math Function2/1 -> Product/2, Sum of Elements3/1  "parallel norton r0 [Ohm]"
  Product/1 -> Sum of Elements2/1  "parallel thevenin voltage [V]"
  Math Function1/1 -> Sum of Elements1/1  "inversed r0 [1/Ohm]"
  Sum of Elements3/1 -> pack thevenin resistance [Ohm]/1
  Sum of Elements2/1 -> pack thevenin voltage [V]/1
  equiv cell voltage [V]/1 -> Divide/1

== system order_reduction_model/electrical model/equivalent circuit/Subsystem ==
  note: Discrete time integrator using the time step
  In1 : Inport
  Memory : Memory
  Sum3 : Sum  Inputs=|++
  Time step : Gain  Gain=conf.time.step
  Out1 : Outport
  wires:
  In1/1 -> Time step/1
  Memory/1 -> Out1/1, Sum3/2  "T"
  Sum3/1 -> Memory/1
  Time step/1 -> Sum3/1

== system order_reduction_model/electrical model/state of charge/Subsystem ==
  note: Discrete time integrator using the time step
  In1 : Inport
  Memory : Memory  InitialCondition=elecInitSOC
  Sum3 : Sum  Inputs=|++
  Time step : Gain  Gain=conf.time.step
  Out1 : Outport
  wires:
  In1/1 -> Time step/1
  Memory/1 -> Out1/1, Sum3/2  "T"
  Sum3/1 -> Memory/1
  Time step/1 -> Sum3/1

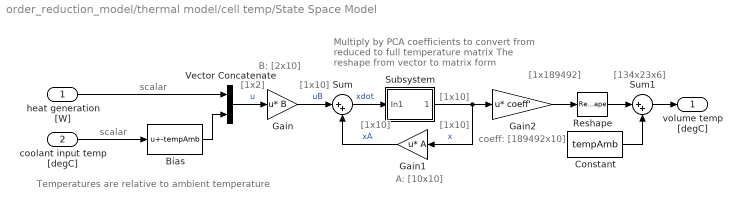
== system order_reduction_model/thermal model/cell temp/State Space Model ==
  note: [1x10]
  note: B: [2x10]
  note: [1x2]
  note: scalar
  note: Multiply by PCA coefficients to convert from reduced to full temperature matrix
      | The reshape from vector to matrix form
  note: Temperatures are relative to ambient temperature
  note: scalar
  note: [1x10]
  note: A: [10x10]
  note: [1x10]
  note: coeff: [189492x10]
  note: [1x189492]
  note: [1x10]
  note: [134x23x6]
  heat generation [W] : Inport
  coolant input temp [degC] : Inport  Port=2
  Bias : Bias  Bias=-tempAmb
  Constant : Constant  Value=tempAmb
  Gain : Gain  Gain=B  Multiplication=Matrix(u*K)
  Gain1 : Gain  Gain=A  Multiplication=Matrix(u*K)
  Gain2 : Gain  Gain=coeff'  Multiplication=Matrix(u*K)
  Reshape : Reshape  OutputDimensionality=Customize  OutputDimensions=thermDims
  Subsystem : Subsystem
      mask Display: disp('DT Int');
  Sum : Sum  Inputs=|++
  Sum1 : Sum  Inputs=|++
  Vector Concatenate : Concatenate
  volume temp [degC] : Outport
  wires:
  heat generation [W]/1 -> Vector Concatenate/1
  coolant input temp [degC]/1 -> Bias/1
  Bias/1 -> Vector Concatenate/2
  Sum/1 -> Subsystem/1(In1)  "xdot"
  Subsystem/1(Out1) -> Gain2/1, Gain1/1  "x"
  Vector Concatenate/1 -> Gain/1  "u"
  Gain/1 -> Sum/1  "uB"
  Gain1/1 -> Sum/2  "xA"
  Gain2/1 -> Reshape/1
  Reshape/1 -> Sum1/1
  Sum1/1 -> volume temp [degC]/1
  Constant/1 -> Sum1/2

== system order_reduction_model/thermal model/cell temp/State Space Model/Subsystem ==
  note: Discrete time integrator using the time step
  In1 : Inport
  Memory : Memory  InitialCondition=zeros(1,10)
  Sum3 : Sum  Inputs=|++
  Time step : Gain  Gain=conf.time.step
  Out1 : Outport
  wires:
  In1/1 -> Time step/1
  Memory/1 -> Out1/1, Sum3/2  "T"
  Sum3/1 -> Memory/1
  Time step/1 -> Sum3/1

== matlab function order_reduction_model/electrical model/cell loading/Cell Loading Function ==
  data: veqMat input; cellCurrent output size=cellsS,cellsP; ibat input; r0Mat input; cellsS parameter; cellsP parameter; elecLoadDenomInds parameter; elecLoadTerm12Inds parameter; elecLoadTerm1Inds parameter; elecLoadTerm2Inds parameter; elecLoadTerm3Inds parameter
function cellCurrent  = cell_loading(veqMat, ibat, r0Mat, cellsS, cellsP, elecLoadDenomInds, elecLoadTerm12Inds, elecLoadTerm1Inds, elecLoadTerm2Inds, elecLoadTerm3Inds)
% Calculate current in each cell
if cellsP == 1
    % All cells take the same current if only in parallel
    term1 = ibat*ones(size(veqMat));   
    term2 = 0; term3 = 0; denom = 1;
elseif cellsP == 2
    % Calculate the current in each cell using pre defined index matrices
    denom = reshape(sum(r0Mat(elecLoadDenomInds)),cellsS,cellsP);
    term1 = veqMat;
    term2 = -reshape(veqMat(elecLoadTerm12Inds),cellsS,cellsP);
    term3 = ibat*reshape(r0Mat(elecLoadTerm12Inds),cellsS,cellsP);
else   
    % Calculate the current in each cell using pre defined index matrices
    denom = reshape(sum(prod(r0Mat(elecLoadDenomInds),2)),cellsS,cellsP);
    term1 = veqMat.*reshape(sum(prod(r0Mat(elecLoadTerm1Inds),2)),cellsS,cellsP);
    term2 = -reshape(sum(veqMat(elecLoadTerm2Inds(:,1,:)).*prod(r0Mat(elecLoadTerm2Inds(:,2:end,:)),2)),cellsS,cellsP);
    term3 = ibat*reshape(prod(r0Mat(elecLoadTerm3Inds)),cellsS,cellsP);
end
cellCurrent = (term1 + term2 + term3)./denom;

== matlab function order_reduction_model/electrical model/cell loading/Cell Loading Function2 ==
  data: veqMat input; cellCurrent output size=seriesCells,parallelCells; powerPack input; r0Mat input; seriesCells parameter; parallelCells parameter; loadDenomInds parameter; loadTerm12Inds parameter; loadTerm1Inds parameter; loadTerm2Inds parameter; loadTerm3Inds parameter; ibat output
function [cellCurrent,ibat] = cell_loading(veqMat,powerPack,r0Mat,seriesCells, parallelCells, loadDenomInds, loadTerm12Inds, loadTerm1Inds, loadTerm2Inds, loadTerm3Inds)
% Find thevenin voltage and resistance
% Individual cell norton - resistance is the same
inMat = veqMat./r0Mat; % Norton current for each cell
% Norton for each set of parallel cells - vector result
inVec = sum(inMat,2); % Norton current for each column
r0MatInv = 1./r0Mat; % Inverse (reciprocal) resistances
rnVec = 1./sum(r0MatInv,2); % Norton resistance for each row
% Final thevenin
vth = sum(rnVec.*inVec); % Thevenin voltage
rth = sum(rnVec); % Thevenin resistance

% Overall current calculation
if vth^2 - 4*rth*powerPack < 0 % Solution is not possible
    % Sets battery current to 0, avoiding error
    ibat = 0;
else
    ibat1 = (vth + sqrt(vth^2 - 4*rth*powerPack))/(2*rth);
    ibat2 = (vth - sqrt(vth^2 - 4*rth*powerPack))/(2*rth);
    ibat = min([ibat1 ibat2]);
end


% Calculate current in each cell
if parallelCells == 1
    % All cells take the same current if only in parallel
    term1 = ibat*ones(size(veqMat));   
    term2 = 0; term3 = 0; denom = 1;
elseif parallelCells == 2
    % Calculate the current in each cell using pre defined index matrices
    denom = reshape(sum(r0Mat(loadDenomInds)),seriesCells,parallelCells);
    term1 = veqMat;
    term2 = -reshape(veqMat(loadTerm12Inds),seriesCells,parallelCells);
    term3 = ibat*reshape(r0Mat(loadTerm12Inds),seriesCells,parallelCells);
else   
    % Calculate the current in each cell using pre defined index matrices
    denom = reshape(sum(prod(r0Mat(loadDenomInds),2)),seriesCells,parallelCells);
    term1 = veqMat.*reshape(sum(prod(r0Mat(loadTerm1Inds),2)),seriesCells,parallelCells);
    term2 = -reshape(sum(veqMat(loadTerm2Inds(:,1,:)).*prod(r0Mat(loadTerm2Inds(:,2:end,:)),2)),seriesCells,parallelCells);
    term3 = ibat*reshape(prod(r0Mat(loadTerm3Inds)),seriesCells,parallelCells);
end
cellCurrent = (term1 + term2 + term3)./denom;

== matlab function order_reduction_model/thermal model/cell temp/map volume temp to cells ==
  data: volTemp input size=thermDims; cellTemp output size=cellsS,cellsP; thermTempInds parameter; cellsS parameter; cellsP parameter
function cellTemp = fcn(volTemp, thermTempInds, cellsS, cellsP)
% Map volume temperatures to cell format for use in electrical model
cellTemp = reshape(mean(volTemp(thermTempInds),1),cellsS,cellsP);
